simulink model "BlackStart_Harness"  (R2025b)
settings: Solver=FixedStepDiscrete  StartTime=0.0  StopTime=20  RelTol=1e-3
PostLoadFcn:
  | BlackStartParam;
values from neighbouring files (symbols this model uses):
  Ts = 5E-5    (= 5e-05)    [BESSGFLParam.m]    (also in BESSGFMParam.m; WindFarmParam.m)
undefined symbols (not defined in the file or in its folder): DiscIntNeverNeededParam
settings Model: Creator=skota  LastModifiedBy=skota

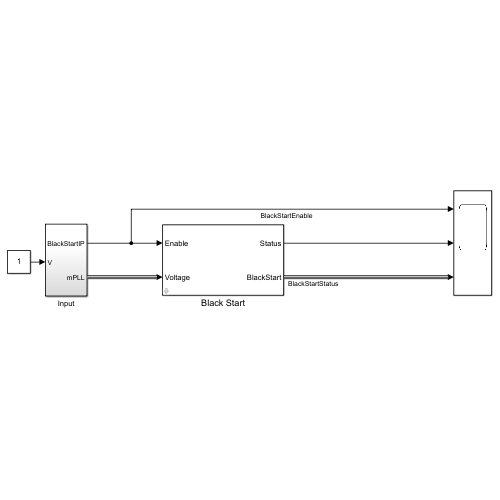
[thumbnail: Simulink's stored preview of the top-level diagram]
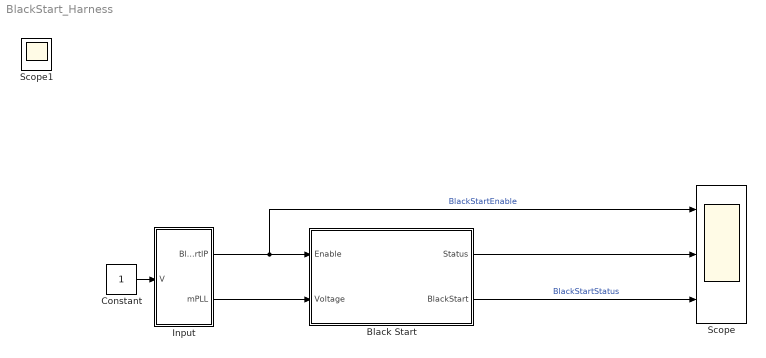
== system BlackStart_Harness ==
  Black Start : Subsystem  mask(BlackStart){referenceFrequency=50, controllerBlackStart=2, voltageLevel1=0.3, voltageLevel2=0.3, voltageLevel3=0.2, delayLevel1=2, delayLevel2=2, delayLevel3=2}
      mask prompts: referenceFrequency "Reference Frequency"; controllerBlackStart "Black Start Time"; voltageLevel1 "Level1"; voltageLevel2 "Level2"; voltageLevel3 "Level3"; delayLevel1 "Delay1"; delayLevel2 "Delay2"; delayLevel3 "Delay3"
      mask help: This block implements the black start logic in the microgrid
      settings: CopyFcn=set_param(gcbh,'LinkStatus','none')
      mask Help: web('BlackStart.html')
      mask DialogControl Container4 Prompt: General
      mask DialogControl Container5 Prompt: Voltage Levels
      mask DialogControl Container6 Prompt: Time Delay
  Constant : Constant
  Input : Subsystem
  Scope : Scope  NumInputPorts=3
      settings: ActiveDisplayYMinimum=-0.12499999999999997  ActiveDisplayYMaximum=1.125
  Scope1 : Scope
      settings: DataLoggingVariableName=ScopeData3
  wires:
  Input/2(mPLL) -> Black Start/2(Voltage)
  Black Start/1(Status) -> Scope/2
  Input/1(BlackStartIP) -> Scope/1, Black Start/1(Enable)  "BlackStartEnable"
  Constant/1 -> Input/1(V)
  Black Start/2(BlackStart) -> Scope/3  "BlackStartStatus"

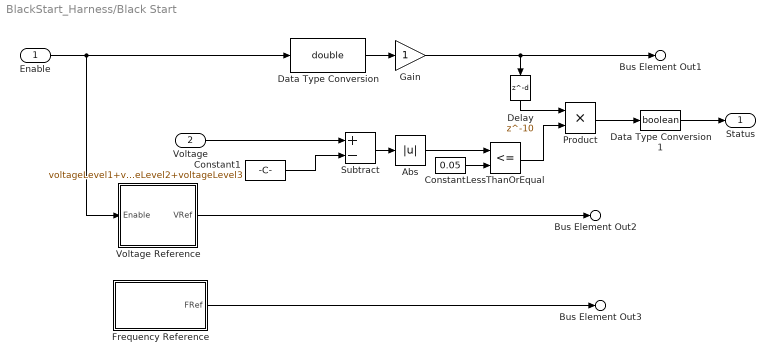
== system BlackStart_Harness/Black Start ==
  Enable : Inport  OutDataTypeStr=boolean
  Voltage : Inport  Port=2
  Abs : Abs  SaturateOnIntegerOverflow=off
  Constant : Constant  Value=0.05
  Constant1 : Constant  Value=voltageLevel1+voltageLevel2+voltageLevel3
  Data Type Conversion : DataTypeConversion  OutDataTypeStr=double  SaturateOnIntegerOverflow=off  RndMeth=Floor
  Data Type Conversion1 : DataTypeConversion  OutDataTypeStr=boolean  SaturateOnIntegerOverflow=off  RndMeth=Floor
  Delay : Delay  DelayLength=10
  Frequency Reference : Subsystem
  Gain : Gain
  LessThanOrEqual : RelationalOperator  Operator=<=  OutDataTypeStr=boolean  RndMeth=Simplest  InputSameDT=off
  Product : Product
  Subtract : Sum  Inputs=+-
  Voltage Reference : Subsystem
  Status : Outport
  Bus Element Out2 : Outport  Port=2  PortName=BlackStart  Element=Vref
  Bus Element Out3 : Outport  Port=2  PortName=BlackStart  Element=Fref
  Bus Element Out1 : Outport  Port=2  PortName=BlackStart  Element=enableCommand
  wires:
  Voltage Reference/1(VRef) -> Bus Element Out2/1
  Data Type Conversion/1 -> Gain/1
  Data Type Conversion1/1 -> Status/1
  Enable/1 -> Voltage Reference/1(Enable), Data Type Conversion/1
  Delay/1 -> Product/1
  Abs/1 -> LessThanOrEqual/1
  Constant1/1 -> Subtract/2
  Product/1 -> Data Type Conversion1/1
  Voltage/1 -> Subtract/1
  Constant/1 -> LessThanOrEqual/2
  LessThanOrEqual/1 -> Product/2
  Frequency Reference/1(FRef) -> Bus Element Out3/1
  Subtract/1 -> Abs/1
  Gain/1 -> Bus Element Out1/1, Delay/1

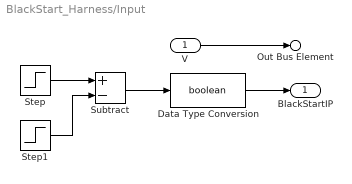
== system BlackStart_Harness/Input ==
  V : Inport
  Data Type Conversion : DataTypeConversion  OutDataTypeStr=boolean  SaturateOnIntegerOverflow=off  RndMeth=Floor
  Step : Step  Time=5  SampleTime=0
  Step1 : Step  Time=14  SampleTime=0
  Subtract : Sum  Inputs=+-
  BlackStartIP : Outport
  Out Bus Element : Outport  Port=2  PortName=mPLL  Element=Island.voltage
  wires:
  V/1 -> Out Bus Element/1
  Data Type Conversion/1 -> BlackStartIP/1
  Subtract/1 -> Data Type Conversion/1
  Step/1 -> Subtract/1
  Step1/1 -> Subtract/2

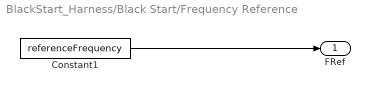
== system BlackStart_Harness/Black Start/Frequency Reference ==
  Constant1 : Constant  Value=referenceFrequency
  FRef : Outport
  wires:
  Constant1/1 -> FRef/1

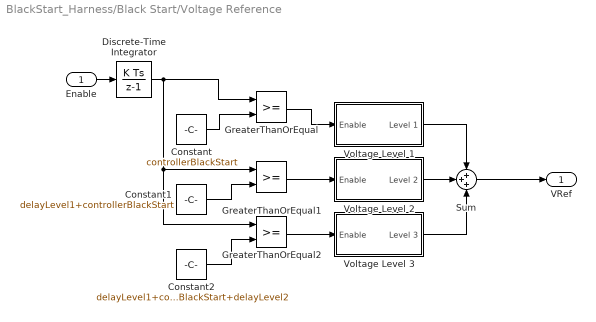
== system BlackStart_Harness/Black Start/Voltage Reference ==
  Enable : Inport
  Constant : Constant  Value=controllerBlackStart
  Constant1 : Constant  Value=delayLevel1+controllerBlackStart
  Constant2 : Constant  Value=delayLevel1+controllerBlackStart+delayLevel2
  Discrete-Time Integrator : DiscreteIntegrator  SampleTime=Ts  OutDataTypeStr=double  ICPrevOutput=DiscIntNeverNeededParam  ICPrevScaledInput=DiscIntNeverNeededParam
  GreaterThanOrEqual : RelationalOperator  OutDataTypeStr=boolean  RndMeth=Simplest  InputSameDT=off
  GreaterThanOrEqual1 : RelationalOperator  OutDataTypeStr=boolean  RndMeth=Simplest  InputSameDT=off
  GreaterThanOrEqual2 : RelationalOperator  OutDataTypeStr=boolean  RndMeth=Simplest  InputSameDT=off
  Sum : Sum  Inputs=+++
  Voltage Level 1 : Subsystem
  Voltage Level 2 : Subsystem
  Voltage Level 3 : Subsystem
  VRef : Outport
  wires:
  Sum/1 -> VRef/1
  Voltage Level 2/1(Level 2) -> Sum/2
  Voltage Level 3/1(Level 3) -> Sum/3
  Voltage Level 1/1(Level 1) -> Sum/1
  GreaterThanOrEqual/1 -> Voltage Level 1/1(Enable)
  GreaterThanOrEqual1/1 -> Voltage Level 2/1(Enable)
  Enable/1 -> Discrete-Time Integrator/1
  Discrete-Time Integrator/1 -> GreaterThanOrEqual2/1, GreaterThanOrEqual1/1, GreaterThanOrEqual/1
  Constant/1 -> GreaterThanOrEqual/2
  Constant1/1 -> GreaterThanOrEqual1/2
  GreaterThanOrEqual2/1 -> Voltage Level 3/1(Enable)
  Constant2/1 -> GreaterThanOrEqual2/2

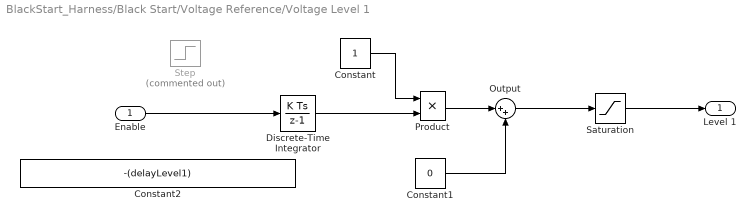
== system BlackStart_Harness/Black Start/Voltage Reference/Voltage Level 1 ==
  Enable : Inport
  Constant : Constant
  Constant1 : Constant  Value=0
  Constant2 : Constant  DisableCoverage=on  Value=-(delayLevel1)  OutDataTypeStr=Inherit: Inherit via back propagation  SampleTime=Ts
  Discrete-Time Integrator : DiscreteIntegrator  SampleTime=Ts  OutDataTypeStr=double  ICPrevOutput=DiscIntNeverNeededParam  ICPrevScaledInput=DiscIntNeverNeededParam
  Output : Sum  Inputs=|++  InputSameDT=on  SaturateOnIntegerOverflow=on  OutDataTypeStr=Inherit: Same as first input
  Product : Product  DisableCoverage=on  InputSameDT=on  SaturateOnIntegerOverflow=on  OutDataTypeStr=Inherit: Same as first input
  Saturation : Saturate  UpperLimit=voltageLevel1  LowerLimit=0
  Step : Step  Commented=on  DisableCoverage=on  Time=controllerBlackStart+delayLevel1  OutDataTypeStr=fixdt('double', 'DataTypeOverride', 'Off')  SampleTime=Ts
  Level 1 : Outport
  wires:
  Discrete-Time Integrator/1 -> Product/2
  Saturation/1 -> Level 1/1
  Product/1 -> Output/1
  Output/1 -> Saturation/1
  Enable/1 -> Discrete-Time Integrator/1
  Constant/1 -> Product/1
  Constant1/1 -> Output/2

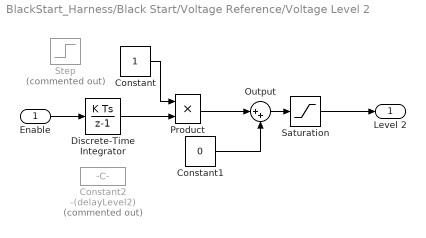
== system BlackStart_Harness/Black Start/Voltage Reference/Voltage Level 2 ==
  Enable : Inport
  Constant : Constant
  Constant1 : Constant  Value=0
  Constant2 : Constant  Commented=on  DisableCoverage=on  Value=-(delayLevel2)  OutDataTypeStr=Inherit: Inherit via back propagation  SampleTime=Ts
  Discrete-Time Integrator : DiscreteIntegrator  SampleTime=Ts  OutDataTypeStr=double  ICPrevOutput=DiscIntNeverNeededParam  ICPrevScaledInput=DiscIntNeverNeededParam
  Output : Sum  Inputs=|++  InputSameDT=on  SaturateOnIntegerOverflow=on  OutDataTypeStr=Inherit: Same as first input
  Product : Product  DisableCoverage=on  InputSameDT=on  SaturateOnIntegerOverflow=on  OutDataTypeStr=Inherit: Same as first input
  Saturation : Saturate  UpperLimit=voltageLevel2  LowerLimit=0
  Step : Step  Commented=on  DisableCoverage=on  Time=delayLevel1+delayLevel2  OutDataTypeStr=fixdt('double', 'DataTypeOverride', 'Off')  SampleTime=Ts
  Level 2 : Outport
  wires:
  Output/1 -> Saturation/1
  Product/1 -> Output/1
  Saturation/1 -> Level 2/1
  Discrete-Time Integrator/1 -> Product/2
  Enable/1 -> Discrete-Time Integrator/1
  Constant/1 -> Product/1
  Constant1/1 -> Output/2

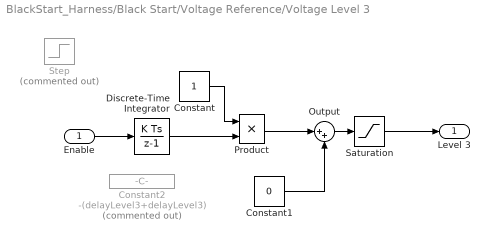
== system BlackStart_Harness/Black Start/Voltage Reference/Voltage Level 3 ==
  Enable : Inport
  Constant : Constant
  Constant1 : Constant  Value=0
  Constant2 : Constant  Commented=on  DisableCoverage=on  Value=-(delayLevel3+delayLevel3)  OutDataTypeStr=Inherit: Inherit via back propagation  SampleTime=Ts
  Discrete-Time Integrator : DiscreteIntegrator  SampleTime=Ts  OutDataTypeStr=double  ICPrevOutput=DiscIntNeverNeededParam  ICPrevScaledInput=DiscIntNeverNeededParam
  Output : Sum  Inputs=|++  InputSameDT=on  SaturateOnIntegerOverflow=on  OutDataTypeStr=Inherit: Same as first input
  Product : Product  DisableCoverage=on  InputSameDT=on  SaturateOnIntegerOverflow=on  OutDataTypeStr=Inherit: Same as first input
  Saturation : Saturate  UpperLimit=voltageLevel3  LowerLimit=0
  Step : Step  Commented=on  DisableCoverage=on  Time=delayLevel1+delayLevel2+delayLevel3  OutDataTypeStr=fixdt('double', 'DataTypeOverride', 'Off')  SampleTime=Ts
  Level 3 : Outport
  wires:
  Discrete-Time Integrator/1 -> Product/2
  Saturation/1 -> Level 3/1
  Product/1 -> Output/1
  Output/1 -> Saturation/1
  Enable/1 -> Discrete-Time Integrator/1
  Constant/1 -> Product/1
  Constant1/1 -> Output/2
